simulink model "simple"  (R2020a)
settings: Solver=VariableStepAuto  StartTime=0.0  StopTime=10.0  RelTol=1e-3
settings Model: Creator=Mertcan  LastModifiedBy=Mertcan

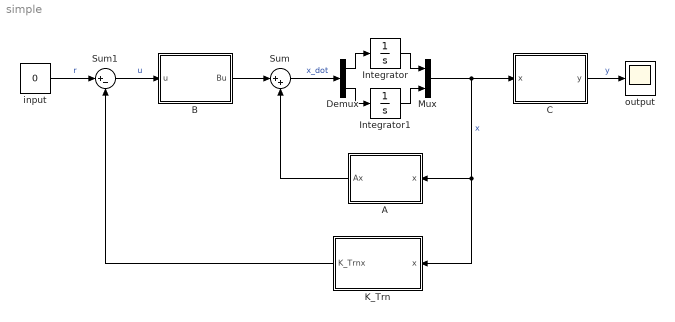
== system simple ==
  A : MATLAB Function  TreatAsAtomicUnit=on
  B : MATLAB Function  TreatAsAtomicUnit=on
  C : MATLAB Function  TreatAsAtomicUnit=on
  Demux : Demux  Outputs=2
  Integrator : Integrator  InitialCondition=1
  Integrator1 : Integrator  InitialCondition=-1
  K_Trn : MATLAB Function  TreatAsAtomicUnit=on
  Mux : Mux  Inputs=2
  Sum : Sum  Inputs=|++
  Sum1 : Sum  Inputs=|+-
  input : Constant  Value=0
  output : Scope
  wires:
  B/1(Bu) -> Sum/1
  Mux/1 -> C/1(x), A/1(x), K_Trn/1(x)  "x"
  Sum/1 -> Demux/1  "x_dot"
  A/1(Ax) -> Sum/2
  K_Trn/1(K_Trnx) -> Sum1/2
  Demux/1 -> Integrator/1
  Demux/2 -> Integrator1/1
  Integrator1/1 -> Mux/2
  Integrator/1 -> Mux/1
  input/1 -> Sum1/1  "r"
  Sum1/1 -> B/1(u)  "u"
  C/1(y) -> output/1  "y"

== matlab function simple/B ==
  data: u input size=1; Bu output size=2
function Bu = B(u)

Bu = [0;u];

== matlab function simple/K_Trn ==
  data: x input size=2; K_Trnx output size=1
function K_Trnx = K_Trn(x)

K_Trnx = k1*x(1) + k2*x(2);

== matlab function simple/C ==
  data: x input size=2; y output size=1
function y = C(x)

C = [1,0];

y = C*x;

== matlab function simple/A ==
  data: x input size=2; Ax output size=2
function Ax = A(x)

Ax = [x(2);-x(1)];
